simulink model "ClosedLoopTestLQR_modular"  (R2025b)
settings: Solver=FixedStepAuto  StartTime=0.0  StopTime=70  FixedStep=Ts  MaxStep=0.015  RelTol=1e-3
StopFcn:
  | stopHeli_allTasks
  | daqreset
model workspace: external: MAT-File (data not in the file)
values from neighbouring files (symbols this model uses):
  Q = diag([Cost_rb Cost_V Cost_I])    [LQR_I.m]
undefined symbols (not defined in the file or in its folder): DAC_lim_u, Discrete, ElevAxisData, l, N, nu, nx, PitchAxisData, q, QN, Time, Ts, U_e_real, x0
libraries: ctrlSharedLib x1, sldrtlib x1
settings Model: VariantConfigurationObject=var_config  Creator=msciola  LastModifiedBy=leeta
settings SolverCC: AlgebraicLoopSolver=TrustRegion
settings DebuggingCC: UnconnectedInputMsg=warning  UnconnectedOutputMsg=warning  UnconnectedLineMsg=warning
settings ModelReferenceCC: EnableRefExpFcnMdlSchedulingChecks=on
settings SFSimCC: CustomCodeUndefinedFunction=UseInterfaceOnly
settings RTWCC: GPUComputeCapability=3.5

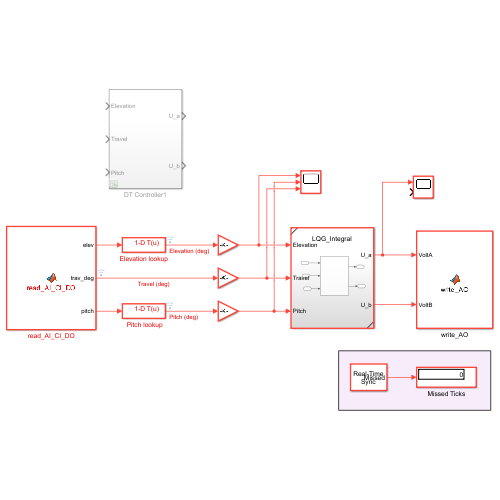
[thumbnail: Simulink's stored preview of the top-level diagram]
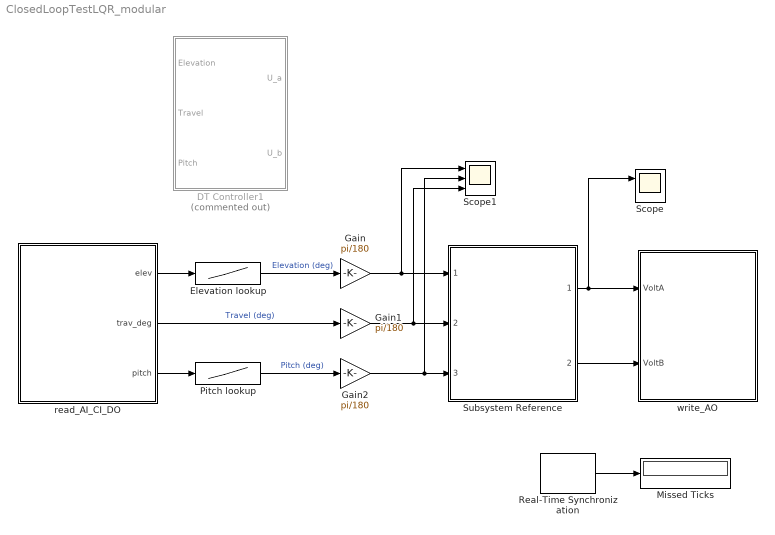
== system ClosedLoopTestLQR_modular ==
  " Pitch lookup" : Lookup_n-D  NumberOfTableDimensions=1  LookupTableObject=PitchAxisData  BreakpointsForDimension1=PitchAxisData.Var2  Table=PitchAxisData.Var1  InternalRulePriority=Speed  RndMeth=Simplest
  DT Controller1 : Subsystem  Commented=on
  Elevation lookup : Lookup_n-D  NumberOfTableDimensions=1  LookupTableObject=PitchAxisData  BreakpointsForDimension1=ElevAxisData.Var2  Table=ElevAxisData.Var1  InternalRulePriority=Speed  RndMeth=Simplest
  Gain : Gain  Gain=pi/180
  Gain1 : Gain  Gain=pi/180
  Gain2 : Gain  Gain=pi/180
  Missed Ticks : Display
  Real-Time Synchronization : sldrtlib/Real-Time Synchronization  SampleTime=Ts  MaxMissedTicks=inf  ShowMissedTicks=on  YieldWhenWaiting=off
  Scope : Scope  NumInputPorts=2
      settings: ActiveDisplayYMinimum=-13.43431784429526  ActiveDisplayYMaximum=17.592246475275068
  Scope1 : Scope  NumInputPorts=3
      settings: ActiveDisplayYMinimum=-0.96320932594779773  ActiveDisplayYMaximum=3.8350465406985323  DataLoggingVariableName=ScopeData2
  Subsystem Reference : Subsystem  ReferencedSubsystem=LQG_Integral
  read_AI_CI_DO : MATLAB Function  TreatAsAtomicUnit=on
  write_AO : MATLAB Function  TreatAsAtomicUnit=on
  wires:
  Real-Time Synchronization/1 -> Missed Ticks/1
  read_AI_CI_DO/3(pitch) -> " Pitch lookup"/1
  read_AI_CI_DO/1(elev) -> Elevation lookup/1
  " Pitch lookup"/1 -> Gain2/1  "Pitch (deg)"
  Elevation lookup/1 -> Gain/1  "Elevation (deg)"
  read_AI_CI_DO/2(trav_deg) -> Gain1/1  "Travel (deg)"
  Gain/1 -> Scope1/1, Subsystem Reference/1
  Gain1/1 -> Scope1/3, Subsystem Reference/2
  Gain2/1 -> Subsystem Reference/3, Scope1/2
  Subsystem Reference/1 -> Scope/1, write_AO/1(VoltA)
  Subsystem Reference/2 -> write_AO/2(VoltB)

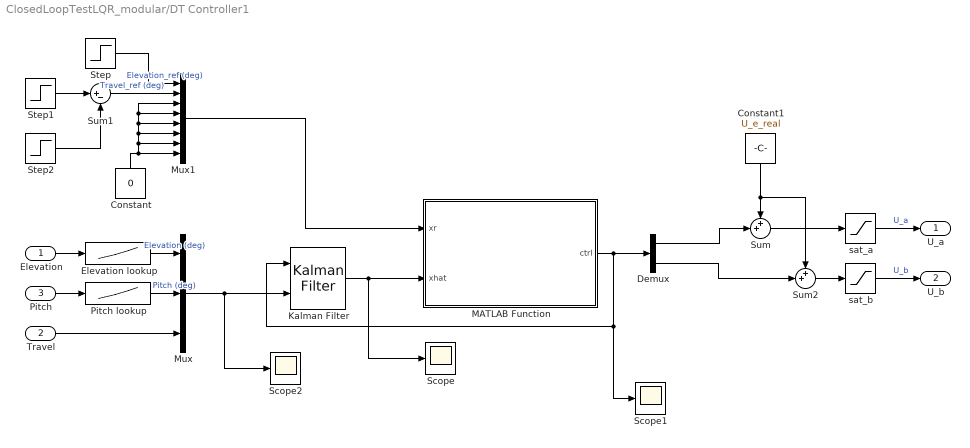
== system ClosedLoopTestLQR_modular/DT Controller1 ==
  Elevation : Inport
  Travel : Inport  Port=2
  Pitch : Inport  Port=3
  " Pitch lookup" : Lookup_n-D  NumberOfTableDimensions=1  LookupTableObject=PitchAxisData  BreakpointsForDimension1=PitchAxisData.Var2  Table=PitchAxisData.Var1  InternalRulePriority=Speed  RndMeth=Simplest
  Constant : Constant  Value=0
  Constant1 : Constant  Value=U_e_real
  Demux : Demux  Outputs=2
  Elevation lookup : Lookup_n-D  NumberOfTableDimensions=1  LookupTableObject=PitchAxisData  BreakpointsForDimension1=ElevAxisData.Var2  Table=ElevAxisData.Var1  InternalRulePriority=Speed  RndMeth=Simplest
  Kalman Filter : ctrlSharedLib/Kalman Filter  TimeDomain=Discrete-Time  UseCurrentEstimator=on  ModelSource=LTI State-Space Variable  ModelSourceVariable=sysdt_comb  A=0.95  B=1  C=1  D=0  NumberOfStates=1  NumberOfInputs=1  NumberOfOutputs=1  InitialEstimateSource=Dialog  X0=x0  P0=10  UseK=off  UseGH=off  NumberOfProcessNoiseInputs=1  G=1  TimeInvariantG=on  H=0  TimeInvariantH=on  Q=0.05  TimeInvariantQ=on  R=1  TimeInvariantR=on  N=0  TimeInvariantN=on  AddInputPort=on  AddEnablePort=off  OutputEstimatedY=off  OutputP=off  Ts=-1
  MATLAB Function : MATLAB Function  TreatAsAtomicUnit=on
  Mux : Mux  Inputs=3
  Mux1 : Mux  Inputs=8
  Scope : Scope
      settings: ActiveDisplayYMinimum=-159.46109872789572  ActiveDisplayYMaximum=590.889478131144  DataLoggingVariableName=ScopeData3
  Scope1 : Scope
      settings: ActiveDisplayYMinimum=-0.669432987929818  ActiveDisplayYMaximum=6.4419123879588991  DataLoggingVariableName=ScopeData4
  Scope2 : Scope
      settings: ActiveDisplayYMinimum=-49.567703006368404  ActiveDisplayYMaximum=46.842206325046462  DataLoggingVariableName=ScopeData3
  Step : Step  Time=0  Before=x0(1)  After=0  SampleTime=Ts
  Step1 : Step  Time=x0(2)  After=0  SampleTime=Ts
  Step2 : Step  Time=0  Before=x0(3)  After=0  SampleTime=Ts
  Sum : Sum  Inputs=++|
  Sum1 : Sum  Inputs=|+-
  Sum2 : Sum  Inputs=++|
  sat_a : Saturate  UpperLimit=DAC_lim_u  LowerLimit=0
  sat_b : Saturate  UpperLimit=DAC_lim_u  LowerLimit=0
  U_a : Outport
  U_b : Outport  Port=2
  wires:
  Step1/1 -> Sum1/1
  Step2/1 -> Sum1/2
  sat_b/1 -> U_b/1  "U_b"
  sat_a/1 -> U_a/1  "U_a"
  Step/1 -> Mux1/1  "Elevation_ref (deg)"
  Sum1/1 -> Mux1/2  "Travel_ref (deg)"
  Travel/1 -> Mux/3
  Mux/1 -> Scope2/1, Kalman Filter/2
  Kalman Filter/1 -> Scope/1, MATLAB Function/2(xhat)
  MATLAB Function/1(ctrl) -> Scope1/1, Kalman Filter/1, Demux/1
  Constant/1 -> Mux1/8, Mux1/6, Mux1/4, Mux1/3, Mux1/5, Mux1/7
  Mux1/1 -> MATLAB Function/1(xr)
  Demux/1 -> Sum/2
  Demux/2 -> Sum2/2
  Sum/1 -> sat_a/1
  Sum2/1 -> sat_b/1
  Constant1/1 -> Sum2/1, Sum/1
  Elevation/1 -> Elevation lookup/1
  " Pitch lookup"/1 -> Mux/2  "Pitch (deg)"
  Pitch/1 -> " Pitch lookup"/1
  Elevation lookup/1 -> Mux/1  "Elevation (deg)"

== matlab function ClosedLoopTestLQR_modular/DT Controller1/MATLAB Function ==
  data: xr input double size=nx; xhat input double size=nx; ctrl output double size=nu; l parameter; u parameter; q parameter; Q parameter; QN parameter; nx parameter; nu parameter; N parameter
function ctrl = mpc_step(xr, xhat, l, u, q, Q, QN, nx, nu, N)

    coder.extrinsic('emosqp')
    % Update OSQP problem
    % Update initial state

    l(1:nx) = -xhat;
    u(1:nx) = -xhat;

    % Update cost for variable xr
    q = [repmat(-Q*xr, N, 1); -QN*xr; zeros(N*nu, 1)];

    emosqp('update_bounds', l, u);
    emosqp('update_lin_cost', q);

    [x, ~, ~, ~, ~] = emosqp('solve'); 

    ctrl = x((N+1)*nx+1:(N+1)*nx+nu);
    % ctrl(1) = ctrl(1) + U_e;
    % ctrl(2) = ctrl(2) + U_e;
end

== matlab function ClosedLoopTestLQR_modular/write_AO ==
  data: VoltA input; VoltB input
function write_AO(VoltA,VoltB)
% The functions from the NI library to write outpus cannot be compiled 
% and we need to use the coder.extrinsic.
% Functions in common to all  
coder.extrinsic('NI_DAQmxCreateTask','NI_DAQmxStartTask', 'assignin');
% Functions to write AO
coder.extrinsic('NI_DAQmxCreateAOVoltageChan','NI_DAQmxWriteAnalogF64',...
    'daq.ni.NIDAQmx.DAQmx_Val_Volts');
%% Configuration
% Specify channel
channelNameAO = {'myDAQ1/ao0','myDAQ1/ao1'};
% make the taskhandle persistent
persistent  taskHandleAO 
% Create and start tasks for each channel
if isempty(taskHandleAO)
    taskHandleAO = NI_DAQmxCreateTask;
    NI_DAQmxCreateAOVoltageChan(taskHandleAO, channelNameAO{1})
    NI_DAQmxCreateAOVoltageChan(taskHandleAO, channelNameAO{2})
    NI_DAQmxStartTask(taskHandleAO);
    assignin('base','taskHandleAO',taskHandleAO);
end
%% Write Digital output
NI_DAQmxWriteAnalogF64(taskHandleAO,[VoltA,VoltB]);
end

== matlab function ClosedLoopTestLQR_modular/read_AI_CI_DO ==
  data: elev output; trav_deg output; pitch output
function [elev,trav_deg,pitch] = read_AI_CI_DO()
% The functions from the NI library to read and write inputs and outpus 
% cannot be compiled and we need to use the coder.extrinsic.
% Functions in common to all 
coder.extrinsic('NI_DAQmxCreateTask','NI_DAQmxStartTask','assignin');
%Functions to read AI
coder.extrinsic('daq.ni.NIDAQmx.DAQmx_Val_Diff','NI_DAQmxCreateAIVoltageChan',...
    'NI_DAQmxReadAnalogF64');
%Functions to read CI
coder.extrinsic('NI_DAQmxCreateCILinEncoderChan','NI_DAQmxReadCounterScalarF64',... 
    'daq.ni.NIDAQmx.DAQmx_Val_X1','daq.ni.NIDAQmx.DAQmx_Val_Ticks');
%Functions to write DO
coder.extrinsic('NI_DAQmxWriteDigitalLines','NI_DAQmxCreateDOChan');

%% Configuration
% Specify channels
channelNameAI = {'myDAQ1/ai0','myDAQ1/ai1'};
channelNameCI = 'myDAQ1/ctr0';
channelNamesDO = {'myDAQ1/Port0/Line5', 'myDAQ1/Port0/Line6','myDAQ1/Port0/Line7'};

% Initialize variables for MATLAB Function block to work
elev = 0;
pitch = 0;
numChannels = 1;
trav = zeros(1, numChannels);
y = zeros(1, numChannels);
% make the taskhandle for each channel persistent
persistent taskHandleAI taskHandleCI taskHandleDO
% Create and start tasks for each channel
if isempty(taskHandleAI)
    taskHandleAI = NI_DAQmxCreateTask;
    NI_DAQmxCreateAIVoltageChan(taskHandleAI, channelNameAI{1}, daq.ni.NIDAQmx.DAQmx_Val_Diff, -10, 10)
    NI_DAQmxCreateAIVoltageChan(taskHandleAI, channelNameAI{2}, daq.ni.NIDAQmx.DAQmx_Val_Diff, -10, 10)
    NI_DAQmxStartTask(taskHandleAI);
    assignin('base','taskHandleAI',taskHandleAI);
end
if isempty(taskHandleCI)
    taskHandleCI = NI_DAQmxCreateTask;
    NI_DAQmxCreateCILinEncoderChan( taskHandleCI, channelNameCI, daq.ni.NIDAQmx.DAQmx_Val_X1, daq.ni.NIDAQmx.DAQmx_Val_Ticks, 1); % Check X4 (Labview) or X1 with Bryn
    NI_DAQmxStartTask(taskHandleCI)
    assignin('base','taskHandleCI',taskHandleCI);
end
if isempty (taskHandleDO)
    taskHandleDO = NI_DAQmxCreateTask;
    for ii = 1:numel(channelNamesDO)
        NI_DAQmxCreateDOChan(taskHandleDO, channelNamesDO{ii});
    end
    %numChannelsDO = NI_DAQmxGetWriteNumChans(taskHandleDO);
    NI_DAQmxStartTask(taskHandleDO)
    assignin('base','taskHandleDO',taskHandleDO);
end
%% Read and write channels
% Write the digital outputs
outputData = [0 1 0];
NI_DAQmxWriteDigitalLines(taskHandleDO, outputData);
% Read analog inputs (elevation and pitch angles)
data = NI_DAQmxReadAnalogF64(taskHandleAI,1,2);
elev = data(1);
pitch = data(2);

% Read the counter encoder input (tavel angle)
y = NI_DAQmxReadCounterScalarF64(taskHandleCI);
% To avoid insignificant numbers in the reading
if y> 2^31
    y = y- 2^32;
end
% Transform the encoder reading into angle degrees between 0 and 360
 trav_deg = y*360/500;
